simulink model "psbseriesload"  (Simulink 6.0)
settings: Solver=ode23s  SolverMode=SingleTasking  StartTime=0.0  StopTime=0.1  RelTol=1e-3  AbsTol=1e-6
libraries: powerlib2 x9
settings Model: Creator=patrice  LastModifiedBy=batserve  ExtModeTrigMode=oneshot  ExtModeArmWhenConnect=off  ExtModeAutoUpdateStatusClock=off
settings DataIOCC: LimitDataPoints=off
settings OptimizationCC: BooleanDataType=off
settings DebuggingCC: SolverPrmCheckMsg=none
settings HardwareCC: TargetUnknown=on
settings RTWCC: TemplateMakefile=grt_unix.tmf

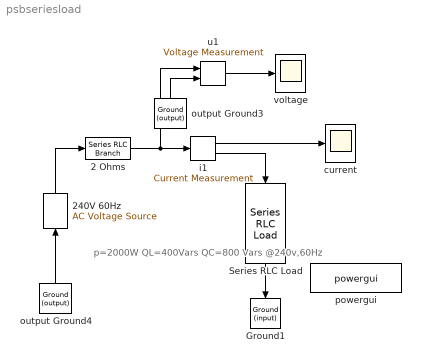
== system psbseriesload ==
  note: p=2000W
      | QL=400Vars
      | QC=800 Vars
      | @240v,60Hz
  2 Ohms : powerlib2/Elements/Series RLC Branch  Tag=PoWeRsYsTeMbLoCk  a=2  b=0  c=inf  mesure=None  PSBOutputType=1
  240V 60Hz : powerlib2/Electrical Sources/AC Voltage Source  Tag=PoWeRsYsTeMbLoCk  Description=source block  Orientation=up  A=240  P=0  F=60  stime=0  mesure=None  PSBOutputType=1
  Ground1 : powerlib2/Connectors/Ground (input)  Tag=PoWeRsYsTeMbLoCk  Orientation=down
  "Series RLC Load " : powerlib2/Elements/Series RLC Load  Tag=PoWeRsYsTeMbLoCk  Orientation=down  a=240  b=60  c=2000  d=400  e=800  mesure=None  PSBOutputType=1
  current : Scope
      settings: TickLabels=on  TimeRange=0.1  YMin=-15  YMax=15  DataFormat=Array
  i1 : powerlib2/Measurements/Current Measurement  Tag=PoWeRsYsTeMmEaSuReMeNt  PSBOutputType=01  PSBequivalent=0
  output Ground3 : powerlib2/Connectors/Ground (output)  Tag=PoWeRsYsTeMbLoCk  Orientation=up  PSBOutputType=1
  output Ground4 : powerlib2/Connectors/Ground (output)  Tag=PoWeRsYsTeMbLoCk  Orientation=up  PSBOutputType=1
  powergui : powerlib2/powergui  matfilesaved=off  Frange=logspace(0,3,50)  Ylog=off  Xlog=off  save=off  variable=ZData  display=off
  u1 : powerlib2/Measurements/Voltage Measurement  Tag=PoWeRsYsTeMmEaSuReMeNt  PSBOutputType=0  PSBequivalent=1
  voltage : Scope
      settings: TickLabels=on  TimeRange=0.1  YMin=-400  YMax=400  DataFormat=Array
  wires:
  240V 60Hz/1 -> 2 Ohms/1
  output Ground4/1 -> 240V 60Hz/1
  output Ground3/1 -> u1/2
  2 Ohms/1 -> u1/1, i1/1
  u1/1 -> voltage/1
  i1/1 -> current/1
  i1/2 -> "Series RLC Load "/1
  "Series RLC Load "/1 -> Ground1/1
